simulink model "TestingCleanPPWithStopACC_Brake"  (R2023a)
settings: Solver=FixedStepAuto  StartTime=0.0  StopTime=inf  FixedStep=0.01  RelTol=1e-3
undefined symbols (not defined in the file): accsubsystem_1_data, x, y, z
libraries: mpcsigdimcheck_private x10, ros2lib x7, robotalgslib x1, mpclib x1, drivingvehiclecontroller x1, slpidlib x1
settings Model: Creator=kartosis  LastModifiedBy=almudhaf.3
settings OptimizationCC: EnhancedBackFolding=on  PassReuseOutputArgsAs=Individual arguments  ZeroExternalMemoryAtStartup=off  ZeroInternalMemoryAtStartup=off  MaxStackSize=64  OptimizeBlockOrder=speed  DifferentSizesBufferReuse=on  OptimizationCustomize=off  EfficientTunableParamExpr=on
settings DebuggingCC: ParameterTunabilityLossMsg=error
settings HardwareCC: ProdBitPerLong=64  ProdHWDeviceType=Intel->x86-64 (Linux 64)
settings SFSimCC: MATLABDynamicMemAlloc=off
settings RTWCC: Description=Embedded Coder  SystemTargetFile=ert.tlc  HardwareBoard=Robot Operating System 2 (ROS 2)  TLCOptions="-aInlineSetEventsForThisBaseRateFcn=TLC_FALSE -aSuppressMultiTaskScheduler=TLC_FALSE  -aRateBasedStepFcn=0"  TemplateMakefile=ert_default_tmf  Toolchain=Colcon Tools  TargetLang=C++
settings CodeAppCC: ForceParamTrailComments=on  IgnoreCustomStorageClasses=off  OperatorAnnotations=on  SimulinkDataObjDesc=on  SFDataObjDesc=on  InsertBlockDesc=on
settings ERTTargetCC: CodeInterfacePackaging=C++ class  RootIOFormat=Structure reference

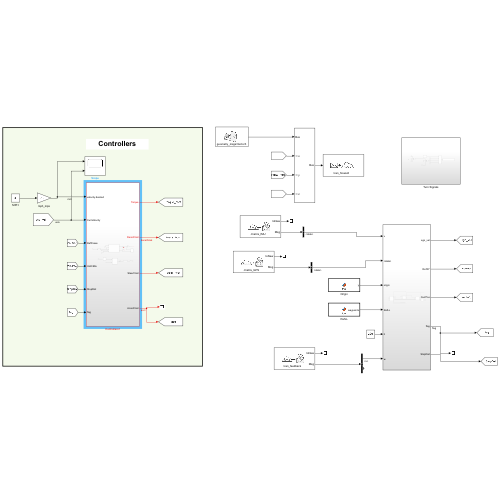
[thumbnail: Simulink's stored preview of the top-level diagram]
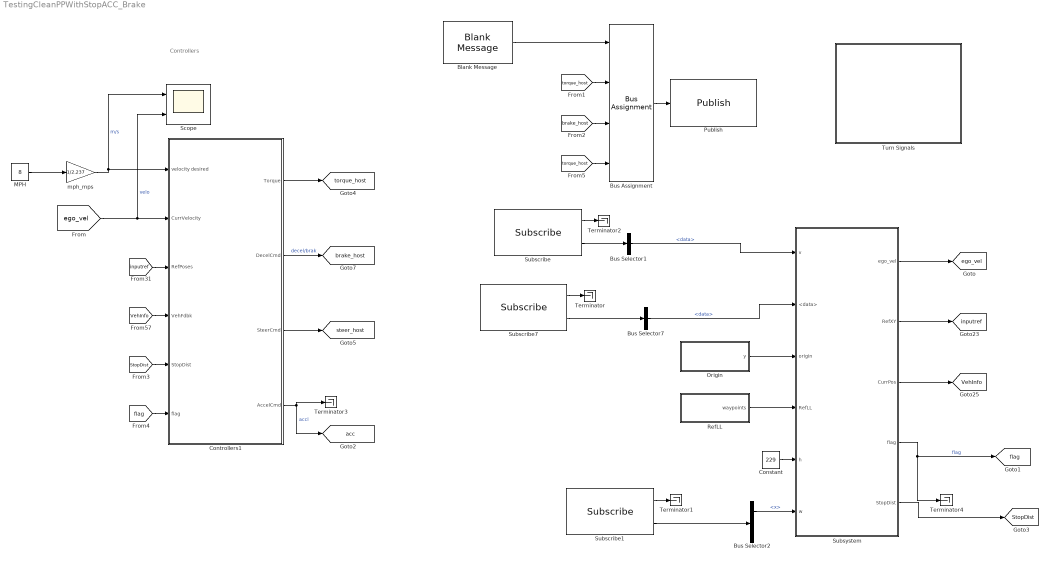
== system TestingCleanPPWithStopACC_Brake ==
  note: Controllers
  Blank Message : ros2lib/Blank Message  messageClass=Message  entityType=geometry_msgs/Vector3  messageType=geometry_msgs/Vector3  SampleTime=0.01
      settings: LibrarySourceBlock=roslib/ROS 2/Blank Message
  Bus Assignment : BusAssignment  AssignedSignals=x,y,z
  Bus Selector1 : BusSelector  OutputSignals=data
  Bus Selector2 : BusSelector  OutputSignals=x,y
  Bus Selector7 : BusSelector  OutputSignals=data
  Constant : Constant  Value=229
  Controllers1 : Subsystem
  MPH : Constant  Value=8
  Origin : MATLAB Function  TreatAsAtomicUnit=on
  Publish : ros2lib/Publish  topicSource=Select from ROS network  topic=/can_forward  messageType=geometry_msgs/Vector3  QOSHistory=Keep last  QOSDepth=1  QOSReliability=Reliable  QOSDurability=Volatile
      settings: LibrarySourceBlock=roslib/ROS 2/Publish
  RefLL : MATLAB Function  TreatAsAtomicUnit=on
  Scope : Scope  NumInputPorts=2
  Subscribe : ros2lib/Subscribe  topicSource=Select from ROS network  topic=/matrix_IMU  messageType=std_msgs/Float64MultiArray  sampleTime=-1  QOSHistory=Keep all  QOSDepth=1  QOSReliability=Reliable  QOSDurability=Volatile
      settings: LibrarySourceBlock=roslib/ROS 2/Subscribe
  Subscribe1 : ros2lib/Subscribe  topicSource=Specify your own  topic=/can_feedback  messageType=geometry_msgs/Vector3  sampleTime=-1  QOSHistory=Keep all  QOSDepth=1  QOSReliability=Reliable  QOSDurability=Volatile
      settings: LibrarySourceBlock=roslib/ROS 2/Subscribe
  Subscribe7 : ros2lib/Subscribe  topicSource=Specify your own  topic=/matrix_GPS  messageType=std_msgs/Float64MultiArray  sampleTime=-1  QOSHistory=Keep all  QOSDepth=1  QOSReliability=Reliable  QOSDurability=Volatile
      settings: LibrarySourceBlock=roslib/ROS 2/Subscribe
  Subsystem : Subsystem
  Terminator{,1..4} (5 alike) : Terminator
  Turn Signals : Subsystem
  mph_mps : Gain  Gain=1/2.237
  tag scope: StopDist=global, VehInfo=global, acc=global, brake_host=global, ego_vel=global, flag=global, inputref=global, steer_host=global, torque_host=global
  wires:
  Blank Message/1 -> Bus Assignment/1
  Bus Assignment/1 -> Publish/1
  Controllers1/1(Torque) -> [torque_host]
  [inputref] -> Controllers1/3(RefPoses)
  [VehInfo] -> Controllers1/4(VehFdbk)
  Controllers1/2(DecelCmd) -> [brake_host]  "decel/brak"
  Controllers1/3(SteerCmd) -> [steer_host]
  Subscribe7/2 -> Bus Selector7/1
  Bus Selector7/1 -> Subsystem/2(<data>)  "<data>"
  Origin/1(y) -> Subsystem/3(origin)
  RefLL/1(waypoints) -> Subsystem/4(RefLL)
  Constant/1 -> Subsystem/5(h)
  Subsystem/1(ego_vel) -> [ego_vel]
  Subsystem/2(RefXY) -> [inputref]
  Bus Selector1/1 -> Subsystem/1(v)  "<data>"
  Subscribe7/1 -> Terminator/1
  Subscribe/2 -> Bus Selector1/1
  Subscribe/1 -> Terminator2/1
  Subsystem/3(CurrPos) -> [VehInfo]
  [ego_vel] -> Controllers1/2(CurrVelocity), Scope/2  "velo"
  mph_mps/1 -> Scope/1, Controllers1/1(velocity desired)  "m/s"
  Subscribe1/1 -> Terminator1/1
  Subscribe1/2 -> Bus Selector2/1
  Bus Selector2/1 -> Subsystem/6(w)  "<x>"
  Controllers1/4(AccelCmd) -> Terminator3/1, [acc]  "accl"
  Subsystem/4(flag) -> Terminator4/1, [flag]  "flag"
  MPH/1 -> mph_mps/1
  [torque_host] -> Bus Assignment/2
  Subsystem/5(StopDist) -> [StopDist]
  [StopDist] -> Controllers1/5(StopDist)
  [flag] -> Controllers1/6(flag)
  [torque_host] -> Bus Assignment/4
  [brake_host] -> Bus Assignment/3

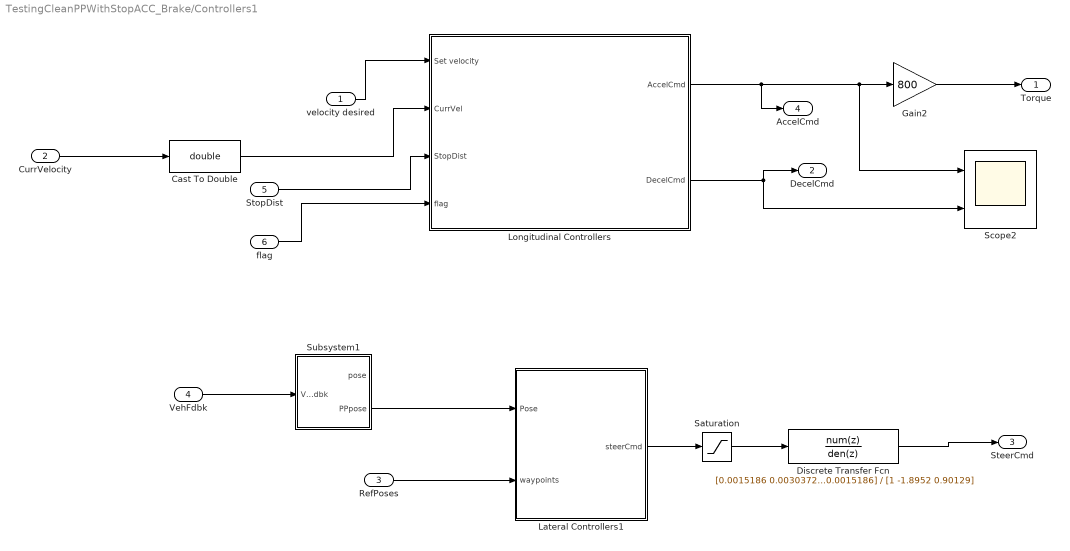
== system TestingCleanPPWithStopACC_Brake/Controllers1 ==
  velocity desired : Inport
  CurrVelocity : Inport  Port=2
  RefPoses : Inport  Port=3
  VehFdbk : Inport  Port=4
  StopDist : Inport  Port=5
  flag : Inport  Port=6
  Cast To Double : DataTypeConversion  OutDataTypeStr=double  SaturateOnIntegerOverflow=off  RndMeth=Floor
  Discrete Transfer Fcn : DiscreteTransferFcn  Numerator=[0.0015186 0.0030372 0.0015186]  Denominator=[1 -1.8952 0.90129]  SampleTime=0.01
  Gain2 : Gain  Gain=800
  Lateral Controllers1 : Subsystem
  Longitudinal Controllers : Subsystem
  Saturation : Saturate  UpperLimit=540  LowerLimit=-540  LinearizeAsGain=off
  Scope2 : Scope  NumInputPorts=2
  Subsystem1 : Subsystem
  Torque : Outport
  DecelCmd : Outport  Port=2
  SteerCmd : Outport  Port=3
  AccelCmd : Outport  Port=4
  wires:
  velocity desired/1 -> Longitudinal Controllers/1(Set velocity)
  Longitudinal Controllers/2(DecelCmd) -> DecelCmd/1, Scope2/2
  Longitudinal Controllers/1(AccelCmd) -> Scope2/1, Gain2/1, AccelCmd/1
  CurrVelocity/1 -> Cast To Double/1
  Subsystem1/2(PPpose) -> Lateral Controllers1/1(Pose)
  VehFdbk/1 -> Subsystem1/1(VehFdbk)
  RefPoses/1 -> Lateral Controllers1/2(waypoints)
  Cast To Double/1 -> Longitudinal Controllers/2(CurrVel)
  Saturation/1 -> Discrete Transfer Fcn/1
  Lateral Controllers1/1(steerCmd) -> Saturation/1
  Discrete Transfer Fcn/1 -> SteerCmd/1
  Gain2/1 -> Torque/1
  StopDist/1 -> Longitudinal Controllers/3(StopDist)
  flag/1 -> Longitudinal Controllers/4(flag)

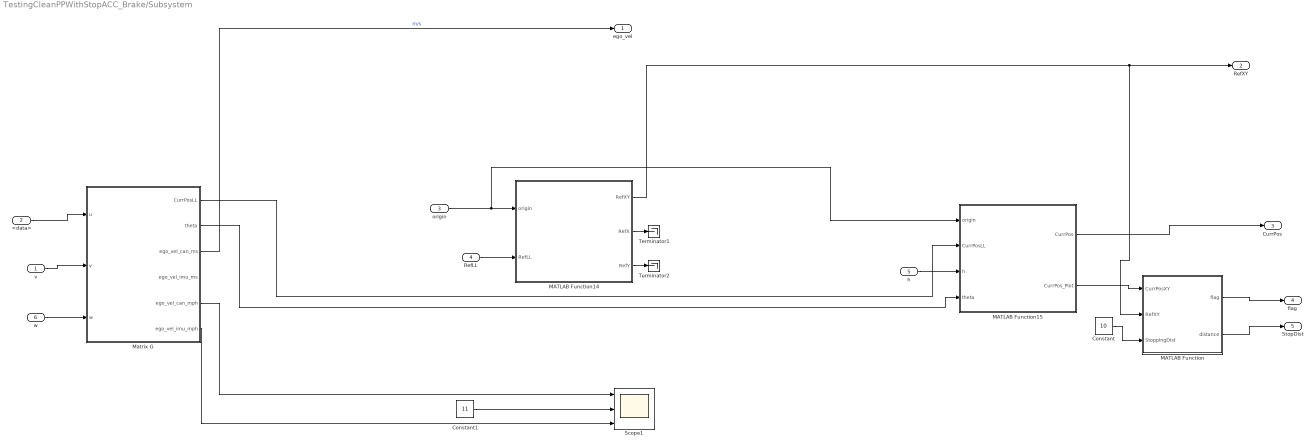
== system TestingCleanPPWithStopACC_Brake/Subsystem ==
  v : Inport
  <data> : Inport  Port=2
  origin : Inport  Port=3
  RefLL : Inport  Port=4
  h : Inport  Port=5
  w : Inport  Port=6
  Constant : Constant  Value=10
  Constant1 : Constant  Value=11
  MATLAB Function : MATLAB Function  TreatAsAtomicUnit=on
  MATLAB Function14 : MATLAB Function  TreatAsAtomicUnit=on
  MATLAB Function15 : MATLAB Function  TreatAsAtomicUnit=on
  Matrix G : MATLAB Function  TreatAsAtomicUnit=on
  Scope1 : Scope  NumInputPorts=3
  Terminator1 : Terminator
  Terminator2 : Terminator
  ego_vel : Outport
  RefXY : Outport  Port=2
  CurrPos : Outport  Port=3
  flag : Outport  Port=4
  StopDist : Outport  Port=5
  wires:
  <data>/1 -> Matrix G/1(u)
  MATLAB Function14/1(RefXY) -> MATLAB Function/2(RefXY), RefXY/1
  MATLAB Function14/3(RefY) -> Terminator2/1
  Matrix G/3(ego_vel_can_ms) -> ego_vel/1  "m/s"
  origin/1 -> MATLAB Function15/1(origin), MATLAB Function14/1(origin)
  Matrix G/2(theta) -> MATLAB Function15/4(theta)
  MATLAB Function15/1(CurrPos) -> CurrPos/1
  RefLL/1 -> MATLAB Function14/2(RefLL)
  h/1 -> MATLAB Function15/3(h)
  Matrix G/1(CurrPosLL) -> MATLAB Function15/2(CurrPosLL)
  MATLAB Function14/2(RefX) -> Terminator1/1
  v/1 -> Matrix G/2(v)
  w/1 -> Matrix G/3(w)
  Constant1/1 -> Scope1/2
  MATLAB Function/1(flag) -> flag/1
  MATLAB Function15/2(CurrPos_Plot) -> MATLAB Function/1(CurrPosXY)
  Matrix G/5(ego_vel_can_mph) -> Scope1/1
  Matrix G/6(ego_vel_imu_mph) -> Scope1/3
  Constant/1 -> MATLAB Function/3(StoppingDist)
  MATLAB Function/2(distance) -> StopDist/1

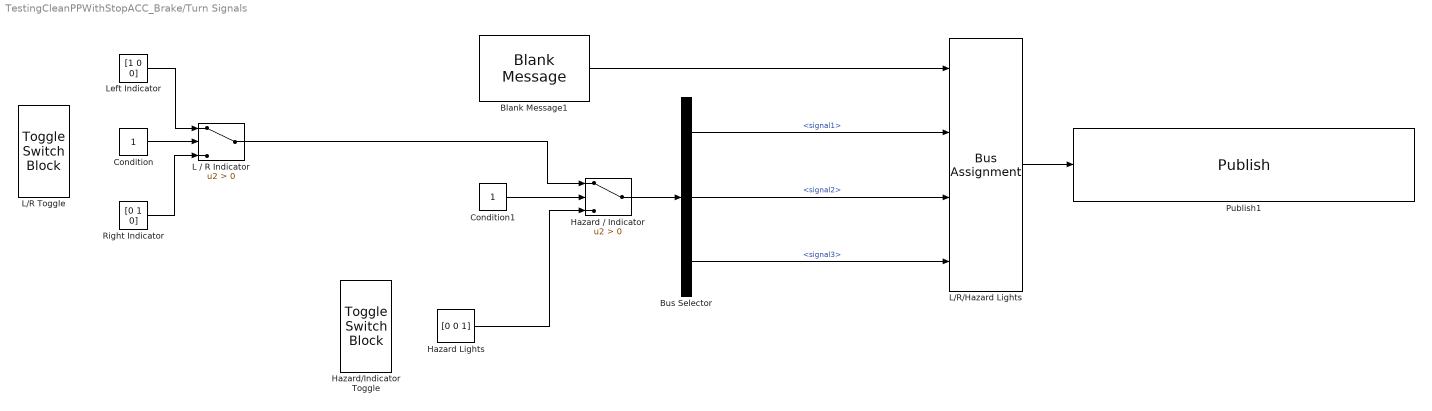
== system TestingCleanPPWithStopACC_Brake/Turn Signals ==
  Blank Message1 : ros2lib/Blank Message  messageClass=Message  entityType=geometry_msgs/Vector3  messageType=geometry_msgs/Vector3  SampleTime=0.01
      settings: LibrarySourceBlock=roslib/ROS 2/Blank Message
  Bus Selector : BusSelector  OutputSignals=signal1,signal2,signal3
  Condition : Constant
  Condition1 : Constant
  Hazard / Indicator : Switch  Criteria=u2 > Threshold  AllowDiffInputSizes=on  SaturateOnIntegerOverflow=off  InputSameDT=off
  Hazard Lights : Constant  Value=[0 0 1]
  Hazard/Indicator Toggle : ToggleSwitchBlock
      settings: Values={{'Off', 'On'}, [0 1]}
  L / R Indicator : Switch  Criteria=u2 > Threshold  SaturateOnIntegerOverflow=off  InputSameDT=off
  L/R Toggle : ToggleSwitchBlock
      settings: Values={{'Off', 'On'}, [0 1]}
  L/R/Hazard Lights : BusAssignment  AssignedSignals=x,y,z
  Left Indicator : Constant  Value=[1 0 0]
  Publish1 : ros2lib/Publish  topicSource=Specify your own  topic=/indicator_lights  messageType=geometry_msgs/Vector3  QOSHistory=Keep last  QOSDepth=1  QOSReliability=Reliable  QOSDurability=Volatile
      settings: LibrarySourceBlock=roslib/ROS 2/Publish
  Right Indicator : Constant  Value=[0 1 0]
  wires:
  Bus Selector/2 -> L/R/Hazard Lights/3  "<signal2>"
  Hazard / Indicator/1 -> Bus Selector/1
  Left Indicator/1 -> L / R Indicator/1
  Bus Selector/3 -> L/R/Hazard Lights/4  "<signal3>"
  Condition/1 -> L / R Indicator/2
  Condition1/1 -> Hazard / Indicator/2
  Right Indicator/1 -> L / R Indicator/3
  L/R/Hazard Lights/1 -> Publish1/1
  Hazard Lights/1 -> Hazard / Indicator/3
  Bus Selector/1 -> L/R/Hazard Lights/2  "<signal1>"
  Blank Message1/1 -> L/R/Hazard Lights/1
  L / R Indicator/1 -> Hazard / Indicator/1

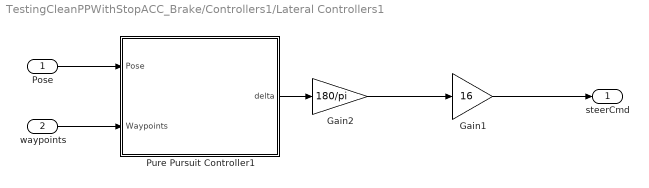
== system TestingCleanPPWithStopACC_Brake/Controllers1/Lateral Controllers1 ==
  Pose : Inport
  waypoints : Inport  Port=2
  Gain1 : Gain  Gain=16
  Gain2 : Gain  Gain=180/pi
  Pure Pursuit Controller1 : Subsystem
  steerCmd : Outport
  wires:
  Pose/1 -> Pure Pursuit Controller1/1(Pose)
  waypoints/1 -> Pure Pursuit Controller1/2(Waypoints)
  Gain2/1 -> Gain1/1
  Gain1/1 -> steerCmd/1
  Pure Pursuit Controller1/1(delta) -> Gain2/1

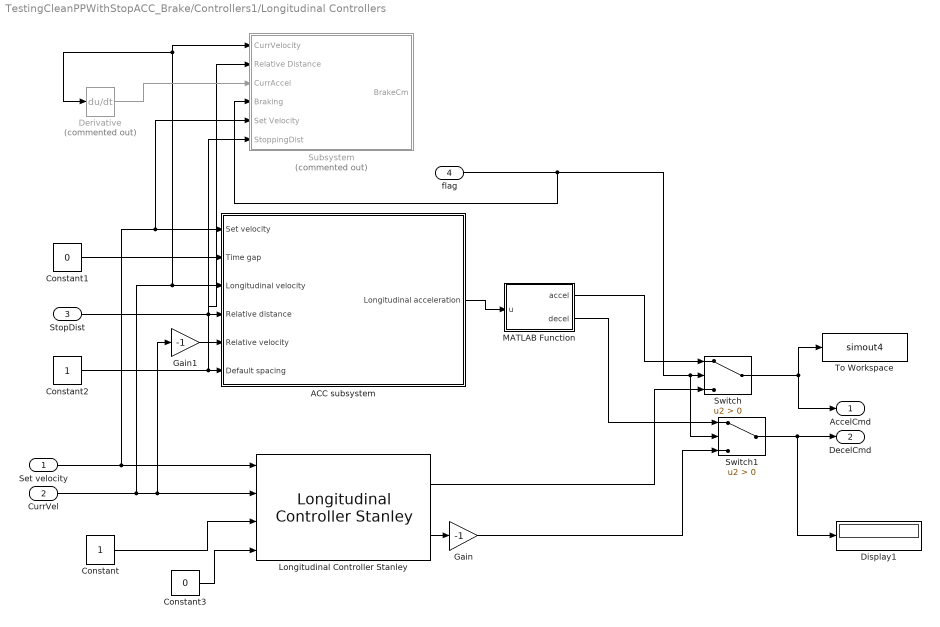
== system TestingCleanPPWithStopACC_Brake/Controllers1/Longitudinal Controllers ==
  Set velocity : Inport
  CurrVel : Inport  Port=2
  StopDist : Inport  Port=3
  flag : Inport  Port=4
  ACC subsystem : Subsystem
      settings: LibrarySourceBlock=mpclib/Automated Driving/Adaptive Cruise Control System
  Constant : Constant
  Constant1 : Constant  Value=0
  Constant2 : Constant
  Constant3 : Constant  Value=0
  Derivative : Derivative  Commented=on
  Display1 : Display
  Gain : Gain  Gain=-1
  Gain1 : Gain  Gain=-1
  Longitudinal Controller Stanley : drivingvehiclecontroller/Longitudinal Controller Stanley  Kp=1.25  Ki=0.12  SampleTime=0.01  MaxAcceleration=2  MaxDeceleration=1.2
  MATLAB Function : MATLAB Function  TreatAsAtomicUnit=on
  Subsystem : Subsystem  Commented=on
  Switch : Switch  Criteria=u2 > Threshold  SaturateOnIntegerOverflow=off  InputSameDT=off
  Switch1 : Switch  Criteria=u2 > Threshold  SaturateOnIntegerOverflow=off  InputSameDT=off
  To Workspace : ToWorkspace  VariableName=simout4  SaveFormat=Timeseries  SampleTime=-1
  AccelCmd : Outport
  DecelCmd : Outport  Port=2
  wires:
  Longitudinal Controller Stanley/2 -> Gain/1
  Set velocity/1 -> Subsystem/5(Set Velocity), ACC subsystem/1(Set velocity), Longitudinal Controller Stanley/1
  Constant3/1 -> Longitudinal Controller Stanley/4
  Constant/1 -> Longitudinal Controller Stanley/3
  CurrVel/1 -> Derivative/1, Subsystem/1(CurrVelocity), ACC subsystem/3(Longitudinal velocity), Gain1/1, Longitudinal Controller Stanley/2
  Constant1/1 -> ACC subsystem/2(Time gap)
  Gain1/1 -> ACC subsystem/5(Relative velocity)
  Constant2/1 -> Subsystem/6(StoppingDist), ACC subsystem/6(Default spacing)
  StopDist/1 -> Subsystem/2(Relative Distance), ACC subsystem/4(Relative distance)
  ACC subsystem/1(Longitudinal acceleration) -> MATLAB Function/1(u)
  flag/1 -> Subsystem/4("Braking "), Switch1/2, Switch/2
  MATLAB Function/1(accel) -> Switch/1
  Longitudinal Controller Stanley/1 -> Switch/3
  Switch/1 -> To Workspace/1, AccelCmd/1
  MATLAB Function/2(decel) -> Switch1/1
  Gain/1 -> Switch1/3
  Switch1/1 -> Display1/1, DecelCmd/1
  Derivative/1 -> Subsystem/3(CurrAccel)

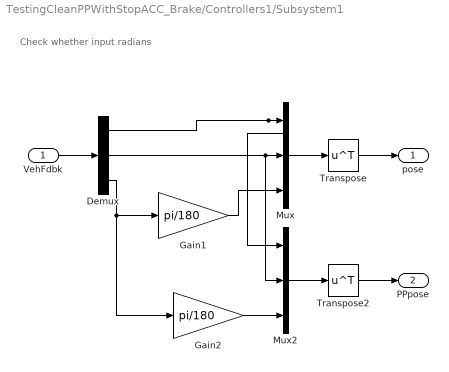
== system TestingCleanPPWithStopACC_Brake/Controllers1/Subsystem1 ==
  note: Check whether input radians
  VehFdbk : Inport
  Demux : Demux  Outputs=3
  Gain1 : Gain  Gain=pi/180
  Gain2 : Gain  Gain=pi/180
  Mux : Mux  Inputs=3
  Mux2 : Mux  Inputs=3
  Transpose : Math  Operator=transpose  SignedPower=on
  Transpose2 : Math  Operator=transpose  SignedPower=on
  pose : Outport
  PPpose : Outport  Port=2
  wires:
  Mux/1 -> Transpose/1
  VehFdbk/1 -> Demux/1
  Gain1/1 -> Mux/3
  Transpose/1 -> pose/1
  Mux2/1 -> Transpose2/1
  Transpose2/1 -> PPpose/1
  Demux/2 -> Mux/2, Mux2/2
  Demux/1 -> Mux2/1, Mux/1
  Demux/3 -> Gain2/1, Gain1/1
  Gain2/1 -> Mux2/3

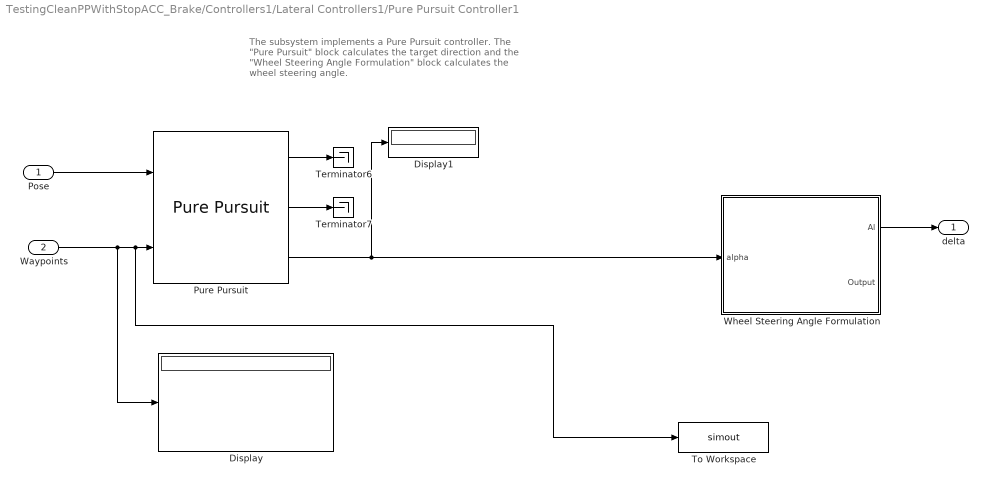
== system TestingCleanPPWithStopACC_Brake/Controllers1/Lateral Controllers1/Pure Pursuit Controller1 ==
  note: The subsystem implements a Pure Pursuit controller. The "Pure Pursuit" block calculates the target direction and the "Wheel Steering Angle Formulation" block calculates the wheel steering angle.
  Pose : Inport
  Waypoints : Inport  Port=2
  Display : Display
  Display1 : Display
  Pure Pursuit : robotalgslib/Pure Pursuit  DesiredLinearVelocity=5  MaxAngularVelocity=1.0  LookaheadDistance=4  TargetDirPort=on  SimulateUsing=Code generation
  Terminator6 : Terminator
  Terminator7 : Terminator
  To Workspace : ToWorkspace  VariableName=simout  SaveFormat=Timeseries  SampleTime=-1
  Wheel Steering Angle Formulation : Subsystem  mask{L=2.865, ld=4}
      mask prompts: L "Bicycle length"; ld "Lookahead distance"
      mask TypeOptions L: Bicycle length/Value
      mask TypeOptions ld: Lookahead distance/Value
      mask Display:
      | image("GeometryMask.png")
      | port_label('input', 1, 'alpha')
      | port_label('output', 1, 'delta')
  delta : Outport
  wires:
  Waypoints/1 -> To Workspace/1, Pure Pursuit/2, Display/1
  Wheel Steering Angle Formulation/1(Al) -> delta/1
  Pure Pursuit/3 -> Wheel Steering Angle Formulation/1(alpha), Display1/1
  Pure Pursuit/2 -> Terminator7/1
  Pose/1 -> Pure Pursuit/1
  Pure Pursuit/1 -> Terminator6/1

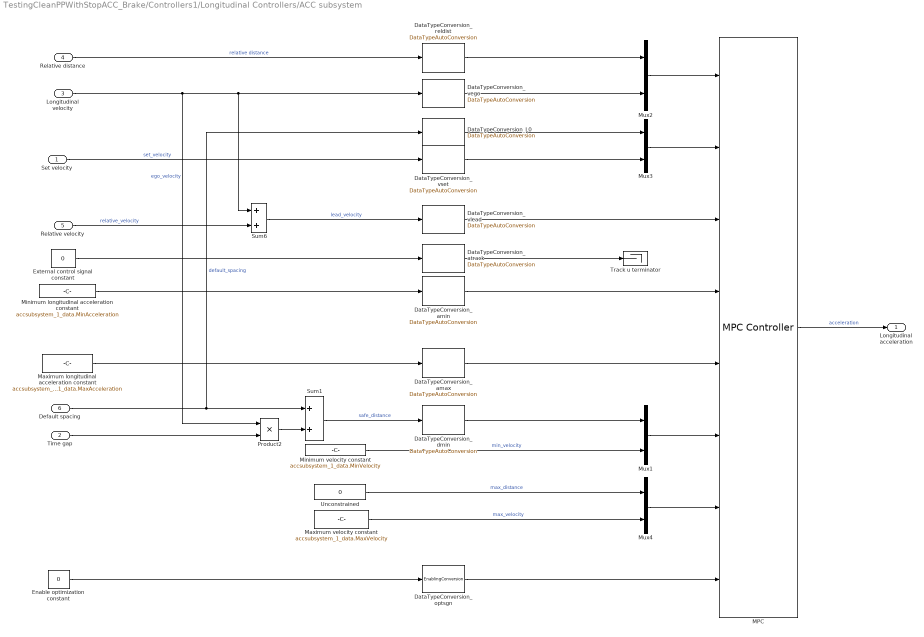
== system TestingCleanPPWithStopACC_Brake/Controllers1/Longitudinal Controllers/ACC subsystem ==
  Set velocity : Inport
  Time gap : Inport  Port=2
  Longitudinal velocity : Inport  Port=3
  Relative distance : Inport  Port=4
  Relative velocity : Inport  Port=5
  Default spacing : Inport  Port=6
  DataTypeConversion_L0 : mpcsigdimcheck_private/DataTypeAutoConversion  datatypestr=accsubsystem_1_data.DataType
      settings: LibrarySourceBlock=mpclib/Automated Driving/Adaptive Cruise Control System/DataTypeConversion_L0
  DataTypeConversion_amax : mpcsigdimcheck_private/DataTypeAutoConversion  datatypestr=accsubsystem_1_data.DataType
      settings: LibrarySourceBlock=mpclib/Automated Driving/Adaptive Cruise Control System/DataTypeConversion_amax
  DataTypeConversion_amin : mpcsigdimcheck_private/DataTypeAutoConversion  datatypestr=accsubsystem_1_data.DataType
      settings: LibrarySourceBlock=mpclib/Automated Driving/Adaptive Cruise Control System/DataTypeConversion_amin
  DataTypeConversion_atrack : mpcsigdimcheck_private/DataTypeAutoConversion  datatypestr=accsubsystem_1_data.DataType
      settings: LibrarySourceBlock=mpclib/Automated Driving/Adaptive Cruise Control System/DataTypeConversion_atrack
  DataTypeConversion_dmin : mpcsigdimcheck_private/DataTypeAutoConversion  datatypestr=accsubsystem_1_data.DataType
      settings: LibrarySourceBlock=mpclib/Automated Driving/Adaptive Cruise Control System/DataTypeConversion_dmin
  DataTypeConversion_optsgn : mpcsigdimcheck_private/EnablingConversion  SystemSampleTime=-1  VariantActivationTime=update diagram  Latency=0  AutoFrameSizeCalculation=off
      settings: LibrarySourceBlock=mpclib/Automated Driving/Adaptive Cruise Control System/DataTypeConversion_optsgn
  DataTypeConversion_reldist : mpcsigdimcheck_private/DataTypeAutoConversion  datatypestr=accsubsystem_1_data.DataType
      settings: LibrarySourceBlock=mpclib/Automated Driving/Adaptive Cruise Control System/DataTypeConversion_reldist
  DataTypeConversion_vego : mpcsigdimcheck_private/DataTypeAutoConversion  datatypestr=accsubsystem_1_data.DataType
      settings: LibrarySourceBlock=mpclib/Automated Driving/Adaptive Cruise Control System/DataTypeConversion_vego
  DataTypeConversion_vlead : mpcsigdimcheck_private/DataTypeAutoConversion  datatypestr=accsubsystem_1_data.DataType
      settings: LibrarySourceBlock=mpclib/Automated Driving/Adaptive Cruise Control System/DataTypeConversion_vlead
  DataTypeConversion_vset : mpcsigdimcheck_private/DataTypeAutoConversion  datatypestr=accsubsystem_1_data.DataType
      settings: LibrarySourceBlock=mpclib/Automated Driving/Adaptive Cruise Control System/DataTypeConversion_vset
  Enable optimization constant : Constant  Value=0  OutDataTypeStr=accsubsystem_1_data.DataType
  External control signal constant : Constant  Value=0  OutDataTypeStr=accsubsystem_1_data.DataType
  MPC : mpclib/MPC Controller  SCDEnableBlockLinearizationSpecification=on  mpcobj=accsubsystem_1_data.Controller  is_multiple=0  enable_value=0  return_u0=off  updateMPCinCallerWorkspace=off  md_inport=on  mv_inport=off  uref_inport=off  return_cost=off  return_mvseq=off  return_qpstatus=off  return_xseq=off  return_state=off  return_ovseq=off  state_inport=off  umin_inport=on  umax_inport=on  ymin_inport=on  ymax_inport=on  cc_inport=off  ywt_inport=off  uwt_inport=off  duwt_inport=off  rhoeps_inport=off  pm_inport=off  MaximumP=10  HorizonChoice=FixedHorizon  n_ts=1  n_p=10  n_mv=1  n_md=2  n_ud=0  n_mo=2  n_uo=0  BlockDataType=double  SampleTimeInherited=off  switch_inport=on
      settings: LibrarySourceBlock=mpclib/Automated Driving/Adaptive Cruise Control System/MPC
  Maximum longitudinal acceleration constant : Constant  Value=accsubsystem_1_data.MaxAcceleration  OutDataTypeStr=accsubsystem_1_data.DataType
  Maximum velocity constant : Constant  Value=accsubsystem_1_data.MaxVelocity  OutDataTypeStr=accsubsystem_1_data.DataType
  Minimum longitudinal acceleration constant : Constant  Value=accsubsystem_1_data.MinAcceleration  OutDataTypeStr=accsubsystem_1_data.DataType
  Minimum velocity constant : Constant  Value=accsubsystem_1_data.MinVelocity  OutDataTypeStr=accsubsystem_1_data.DataType
  Mux{1..4} (4 alike) : Mux  Inputs=[1 1]
  Product2 : Product
  Sum1 : Sum
  Sum6 : Sum
  Track u terminator : Terminator
  Unconstrained : Constant  Value=0  OutDataTypeStr=accsubsystem_1_data.DataType
  Longitudinal acceleration : Outport  PortDimensions=1  VectorParamsAs1DForOutWhenUnconnected=off
  wires:
  DataTypeConversion_atrack/1 -> Track u terminator/1
  External control signal constant/1 -> DataTypeConversion_atrack/1
  DataTypeConversion_optsgn/1 -> MPC/8
  Enable optimization constant/1 -> DataTypeConversion_optsgn/1
  Unconstrained/1 -> Mux4/1  "max_distance"
  Maximum velocity constant/1 -> Mux4/2  "max_velocity"
  Mux4/1 -> MPC/7
  Maximum longitudinal acceleration constant/1 -> DataTypeConversion_amax/1
  Minimum longitudinal acceleration constant/1 -> DataTypeConversion_amin/1
  Set velocity/1 -> DataTypeConversion_vset/1  "set_velocity"
  Time gap/1 -> Product2/2
  DataTypeConversion_vego/1 -> Mux2/2
  DataTypeConversion_reldist/1 -> Mux2/1
  DataTypeConversion_vset/1 -> Mux3/2
  DataTypeConversion_L0/1 -> Mux3/1
  DataTypeConversion_vlead/1 -> MPC/3
  DataTypeConversion_dmin/1 -> Mux1/1
  DataTypeConversion_amin/1 -> MPC/4
  DataTypeConversion_amax/1 -> MPC/5
  Mux1/1 -> MPC/6
  Sum1/1 -> DataTypeConversion_dmin/1  "safe_distance"
  Minimum velocity constant/1 -> Mux1/2  "min_velocity"
  Product2/1 -> Sum1/2
  MPC/1 -> Longitudinal acceleration/1  "acceleration"
  Relative velocity/1 -> Sum6/2  "relative_velocity"
  Relative distance/1 -> DataTypeConversion_reldist/1  "relative distance"
  Longitudinal velocity/1 -> Sum6/1, DataTypeConversion_vego/1, Product2/1  "ego_velocity"
  Mux3/1 -> MPC/2
  Mux2/1 -> MPC/1
  Default spacing/1 -> Sum1/1, DataTypeConversion_L0/1  "default_spacing"
  Sum6/1 -> DataTypeConversion_vlead/1  "lead_velocity"

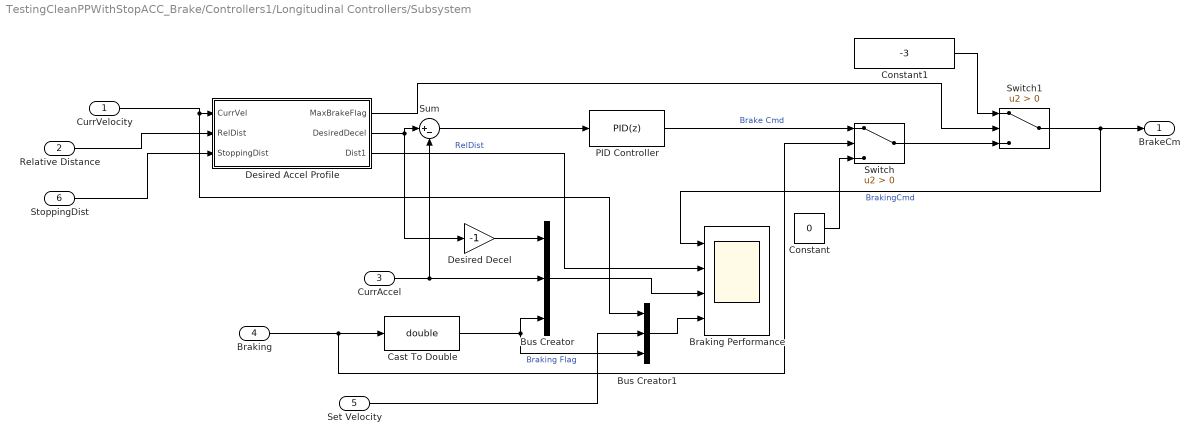
== system TestingCleanPPWithStopACC_Brake/Controllers1/Longitudinal Controllers/Subsystem ==
  CurrVelocity : Inport
  Relative Distance : Inport  Port=2
  CurrAccel : Inport  Port=3
  "Braking " : Inport  Port=4
  Set Velocity : Inport  Port=5
  StoppingDist : Inport  Port=6
  Braking Performance : Scope  NumInputPorts=4
  Bus Creator : BusCreator  Inputs=3
  Bus Creator1 : BusCreator  Inputs=3
  Cast To Double : DataTypeConversion  OutDataTypeStr=double  SaturateOnIntegerOverflow=off  RndMeth=Floor
  Constant : Constant  Value=0
  Constant1 : Constant  Value=-3
  Desired Accel Profile : MATLAB Function  TreatAsAtomicUnit=on
  Desired Decel : Gain  Gain=-1
  PID Controller : slpidlib/PID Controller  Controller=PID  Form=Parallel  TimeDomain=Discrete-time  UseExternalTs=off  SampleTime=0.01  IntegratorMethod=Forward Euler  FilterMethod=Forward Euler  ControllerParametersSource=internal  P=0.05*20  I=0.01*10  UseKiTs=off  D=0  N=100  UseFilter=on  TunerSelectOption=Transfer Function Based (PID Tuner App)  InitialConditionSource=internal  InitialConditionForIntegrator=0  InitialConditionForFilter=0  DifferentiatorICPrevScaledInput=0  ExternalReset=none  TrackingMode=off  Kt=1  LimitOutput=on  SatLimitsSource=internal  UpperSaturationLimit=3  LowerSaturationLimit=-3  LinearizeAsGain=on  AntiWindupMode=none  Kb=1  LimitIntegrator=off  UpperIntegratorSaturationLimit=inf  LowerIntegratorSaturationLimit=-inf  POutMin=[]  POutMax=[]  IOutMin=[]  IOutMax=[]  DOutMin=[]  DOutMax=[]  NOutMin=[]  NOutMax=[]  SumOutMin=[]  SumOutMax=[]  SaturationOutMin=[]  SaturationOutMax=[]  PParamMin=[]  PParamMax=[]  IParamMin=[]  IParamMax=[]  DParamMin=[]  DParamMax=[]  NParamMin=[]  NParamMax=[]  KbParamMin=[]  KbParamMax=[]  KtParamMin=[]  KtParamMax=[]  KbOutMin=[]  KbOutMax=[]  KtOutMin=[]  KtOutMax=[]  IntegratorOutMin=[]  IntegratorOutMax=[]  FilterOutMin=[]  FilterOutMax=[]  SumI1OutMin=[]  SumI1OutMax=[]  SumI2OutMin=[]  SumI2OutMax=[]  SumI3OutMin=[]  SumI3OutMax=[]  SumI4OutMin=[]  SumI4OutMax=[]  SumDOutMin=[]  SumDOutMax=[]  DifferentiatorOutMin=[]  DifferentiatorOutMax=[]  FilterDiffOutCoefMin=[]  FilterDiffOutCoefMax=[]  ReciprocalOutMin=[]  ReciprocalOutMax=[]  SumDenOutMin=[]  SumDenOutMax=[]  SumNumOutMin=[]  SumNumOutMax=[]  DivideOutMin=[]  DivideOutMax=[]  UdiffTsProdOutMin=[]  UdiffTsProdOutMax=[]  NTsProdOutMin=[]  NTsProdOutMax=[]  UintegralTsProdOutMin=[]  UintegralTsProdOutMax=[]  UngainTsProdOutMin=[]  UngainTsProdOutMax=[]  ClampingZeroOutDataTypeStr=Inherit: Inherit via back propagation  ClampingZeroOutMin=[]  ClampingZeroOutMax=[]  FilterDenConstantOutDataTypeStr=Inherit: Inherit via back propagation  FilterDenConstantOutMin=[]  FilterDenConstantOutMax=[]  PCopyOutDataTypeStr=Inherit: Inherit via back propagation  PCopyOutMin=[]  PCopyOutMax=[]  NCopyOutDataTypeStr=Inherit: Inherit via back propagation  NCopyOutMin=[]  NCopyOutMax=[]  IntegratorContinuousStateAttributes=''  IntegratorStateMustResolveToSignalObject=off  IntegratorRTWStateStorageClass=Auto  FilterContinuousStateAttributes=''  FilterStateMustResolveToSignalObject=off  FilterRTWStateStorageClass=Auto  ParallelPVariant=InternalParameters  IdealPVariant=Disabled  IVariant=InternalParameters  DVariant=InternalParameters  IntegratorVariant=Discrete  SatVariant=Enabled  AWVariant=Passthrough  PCopyVariant=Disabled  TRVariant=Disabled  FdbkBlocksVariant=Forward  IdealPFdbkVariant=Disabled  SatFdbkVariant=Disabled  DerivativeFilterVariant=ForwardEulerFilter  NVariant=InternalParameters  NCopyVariant=Disabled  FilterICVariant=InternalICsFilter  IntegratorICVariant=InternalICs  ExternalResetVariant=Disabled  TRSumVariant=Passthrough  SumFdbkVariant=Disabled  SumVariant=Sum_PID  TsampFilterVariant=InternalTs  TsampNgainVariant=Passthrough  TsampIntegralVariant=Disabled_SignalSpec  ExternalSaturationOutDataTypeStr=Inherit: Same as second input
  Sum : Sum  Inputs=|+-
  Switch : Switch  Criteria=u2 > Threshold  SaturateOnIntegerOverflow=off  InputSameDT=off
  Switch1 : Switch  Criteria=u2 > Threshold  SaturateOnIntegerOverflow=off  InputSameDT=off
  BrakeCm : Outport
  wires:
  Relative Distance/1 -> Desired Accel Profile/2(RelDist)
  CurrVelocity/1 -> Bus Creator1/1, Desired Accel Profile/1(CurrVel)
  Sum/1 -> PID Controller/1
  Desired Accel Profile/2(DesiredDecel) -> Sum/1, Desired Decel/1
  "Braking "/1 -> Cast To Double/1, Switch/2
  PID Controller/1 -> Switch/1  "Brake Cmd"
  CurrAccel/1 -> Bus Creator/2, Sum/2
  Desired Decel/1 -> Bus Creator/1
  Constant/1 -> Switch/3
  Switch1/1 -> BrakeCm/1, Braking Performance/1  "BrakingCmd"
  Bus Creator/1 -> Braking Performance/3
  Cast To Double/1 -> Bus Creator1/3, Bus Creator/3  "Braking Flag"
  Desired Accel Profile/3(Dist1) -> Braking Performance/2  "RelDist"
  Switch/1 -> Switch1/3
  Constant1/1 -> Switch1/1
  Desired Accel Profile/1(MaxBrakeFlag) -> Switch1/2
  Bus Creator1/1 -> Braking Performance/4
  Set Velocity/1 -> Bus Creator1/2
  StoppingDist/1 -> Desired Accel Profile/3(StoppingDist)

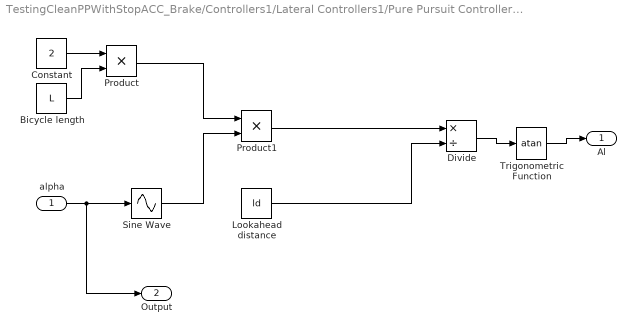
== system TestingCleanPPWithStopACC_Brake/Controllers1/Lateral Controllers1/Pure Pursuit Controller1/Wheel Steering Angle Formulation ==
  alpha : Inport
  Bicycle length : Constant  Value=L
  Constant : Constant  Value=2
  Divide : Product  Inputs=*/
  Lookahead distance : Constant  Value=ld
  Product : Product
  Product1 : Product
  Sine Wave : Sin  TimeSource=Use external signal  SampleTime=0
  Trigonometric Function : Trigonometry  Operator=atan
  Al : Outport
  Output : Outport  Port=2
  wires:
  Sine Wave/1 -> Product1/2
  Bicycle length/1 -> Product/2
  Constant/1 -> Product/1
  Product1/1 -> Divide/1
  Product/1 -> Product1/1
  Divide/1 -> Trigonometric Function/1
  Trigonometric Function/1 -> Al/1
  alpha/1 -> Output/1, Sine Wave/1
  Lookahead distance/1 -> Divide/2

== matlab function TestingCleanPPWithStopACC_Brake/RefLL ==
  data: waypoints output
function waypoints = fcn()


waypoints = [39.99806227837	-83.03238507155	229
39.99806225176	-83.03238507514	229
39.9980622151	-83.03238507952	229
39.99806216774	-83.03238508483	229
39.99806210916	-83.0323850914	229
39.9980620386	-83.03238509932	229
39.99806195496	-83.03238510834	229
39.99806185794	-83.03238511771	229
39.99806174741	-83.03238512699	229
39.99806162342	-83.03238513722	229
39.99806148606	-83.03238514889	229
39.9980613351	-83.03238516134	229
39.99806117106	-83.03238517433	229
39.99806099373	-83.03238518809	229
39.99806080287	-83.03238520311	229
39.99806059877	-83.03238521974	229
39.9980603816	-83.03238523758	229
39.99806015088	-83.03238525624	229
39.99805990597	-83.03238527514	229
39.99805964671	-83.03238529435	229
39.99805937279	-83.03238531348	229
39.99805908445	-83.03238533236	229
39.99805878124	-83.03238535135	229
39.99805846301	-83.0323853721	229
39.99805813043	-83.03238539447	229
39.99805778345	-83.03238541821	229
39.99805742217	-83.03238544562	229
39.99805704525	-83.03238547719	229
39.99805665066	-83.03238551184	229
39.99805623779	-83.03238554698	229
39.99805580651	-83.03238558132	229
39.99805535566	-83.03238561318	229
39.99805488245	-83.03238564368	229
39.99805438579	-83.0323856757	229
39.99805386398	-83.03238570799	229
39.99805331699	-83.03238573957	229
39.99805274668	-83.03238577085	229
39.99805215422	-83.03238580623	229
39.99805153901	-83.03238584858	229
39.99805090072	-83.03238589397	229
39.99805023847	-83.03238593501	229
39.99804955387	-83.0323859732	229
39.99804884854	-83.03238600929	229
39.99804812134	-83.03238604341	229
39.99804736942	-83.03238607335	229
39.99804659222	-83.03238609894	229
39.99804579135	-83.03238612215	229
39.99804496763	-83.0323861475	229
39.99804412175	-83.03238617519	229
39.99804325484	-83.03238620332	229
39.99804236657	-83.032386228	229
39.99804145321	-83.03238625152	229
39.99804051343	-83.032386277	229
39.99803954941	-83.03238630202	229
39.9980385642	-83.03238632304	229
39.9980375606	-83.03238633651	229
39.99803653652	-83.03238634697	229
39.99803548964	-83.03238635868	229
39.99803442351	-83.03238637053	229
39.9980333402	-83.03238638456	229
39.99803223852	-83.03238640484	229
39.99803111484	-83.03238642781	229
39.99802996541	-83.0323864486	229
39.99802879006	-83.03238647172	229
39.99802759101	-83.03238649686	229
39.99802637196	-83.03238652146	229
39.99802513502	-83.03238654417	229
39.99802387934	-83.03238656564	229
39.99802260234	-83.032386585	229
39.99802130181	-83.03238660287	229
39.99801998372	-83.03238661609	229
39.99801864897	-83.0323866234	229
39.99801729425	-83.03238662973	229
39.99801591803	-83.03238663905	229
39.99801452252	-83.03238665271	229
39.99801311009	-83.03238666735	229
39.99801167682	-83.03238667923	229
39.99801021795	-83.03238668921	229
39.99800873742	-83.03238671672	229
39.99800724147	-83.03238675343	229
39.9980057318	-83.03238678991	229
39.99800420585	-83.03238682836	229
39.99800266269	-83.03238687154	229
39.99800110662	-83.032386922	229
39.99799954247	-83.03238697846	229
39.99799796658	-83.03238703209	229
39.99799637829	-83.03238708819	229
39.99799477883	-83.03238714956	229
39.99799317104	-83.0323872162	229
39.99799155708	-83.03238728636	229
39.99798993813	-83.03238735626	229
39.99798831859	-83.03238743124	229
39.99798670493	-83.03238751066	229
39.99798509358	-83.03238761542	229
39.9979834807	-83.0323877503	229
39.99798186778	-83.03238789974	229
39.99798025748	-83.03238805807	229
39.99797865179	-83.03238822672	229
39.99797704903	-83.03238840551	229
39.99797544282	-83.03238859589	229
39.99797383264	-83.03238880248	229
39.99797222769	-83.03238902288	229
39.99797062788	-83.03238924809	229
39.9979690293	-83.03238948477	229
39.99796743185	-83.03238974006	229
39.99796583588	-83.0323900133	229
39.9979642362	-83.03239029449	229
39.99796263389	-83.03239057328	229
39.99796103244	-83.0323908433	229
39.99795942781	-83.03239109745	229
39.99795781729	-83.03239132289	229
39.99795620105	-83.03239152875	229
39.99795457923	-83.03239173027	229
39.99795295492	-83.03239193247	229
39.99795132891	-83.03239214768	229
39.99794969932	-83.03239238496	229
39.99794806376	-83.03239264698	229
39.99794642222	-83.03239292936	229
39.99794478006	-83.03239322594	229
39.99794313768	-83.03239353257	229
39.9979414933	-83.03239384218	229
39.99793984742	-83.03239414331	229
39.99793819886	-83.03239443095	229
39.99793655178	-83.03239470689	229
39.99793491169	-83.03239496597	229
39.99793327721	-83.03239520892	229
39.99793165059	-83.03239545168	229
39.9979300343	-83.03239571043	229
39.99792842977	-83.0323959992	229
39.99792683979	-83.03239632589	229
39.9979252643	-83.03239668805	229
39.99792370386	-83.03239708278	229
39.99792216401	-83.03239751642	229
39.9979206462	-83.0323979888	229
39.99791914359	-83.03239848642	229
39.99791764595	-83.03239900233	229
39.99791615186	-83.03239953319	229
39.99791466259	-83.03240007282	229
39.99791317524	-83.03240062214	229
39.99791169074	-83.03240118781	229
39.99791021889	-83.0324017789	229
39.99790876832	-83.03240240037	229
39.99790734031	-83.03240305497	229
39.9979059366	-83.03240375108	229
39.99790455697	-83.03240449129	229
39.99790319965	-83.03240526838	229
39.9979018623	-83.03240607819	229
39.99790054388	-83.0324069275	229
39.99789924017	-83.03240780389	229
39.99789795049	-83.0324086981	229
39.99789667841	-83.03240961142	229
39.99789542324	-83.03241054286	229
39.99789418065	-83.03241147988	229
39.99789295424	-83.03241244086	229
39.99789174752	-83.03241344165	229
39.99789056469	-83.03241449101	229
39.99788941669	-83.03241558983	229
39.99788830671	-83.03241672758	229
39.99788723077	-83.03241790049	229
39.99788618145	-83.0324191005	229
39.99788515923	-83.0324203259	229
39.99788416924	-83.03242157149	229
39.99788321561	-83.03242283345	229
39.99788229438	-83.03242411282	229
39.99788140433	-83.03242541542	229
39.99788054065	-83.03242674735	229
39.99787969403	-83.03242809984	229
39.99787885465	-83.03242946278	229
39.99787802132	-83.03243083544	229
39.9978772039	-83.03243222385	229
39.99787641925	-83.03243363939	229
39.99787567528	-83.03243508332	229
39.99787496988	-83.0324365466	229
39.99787429569	-83.03243802253	229
39.99787365269	-83.0324395127	229
39.99787304377	-83.03244102356	229
39.99787246485	-83.03244254724	229
39.99787190846	-83.03244407586	229
39.99787137491	-83.03244561086	229
39.99787086386	-83.03244715503	229
39.99787037513	-83.0324487089	229
39.99786991211	-83.03245027402	229
39.99786948354	-83.03245185647	229
39.99786908916	-83.03245345588	229
39.99786871729	-83.03245506829	229
39.9978683647	-83.03245669359	229
39.99786803715	-83.03245833968	229
39.99786773632	-83.03246000806	229
39.99786745744	-83.03246169633	229
39.99786719281	-83.03246340902	229
39.99786693468	-83.03246514706	229
39.99786667599	-83.03246690344	229
39.99786642418	-83.0324686747	229
39.99786618854	-83.03247046119	229
39.99786597319	-83.03247226404	229
39.99786577648	-83.03247408263	229
39.99786560434	-83.03247591964	229
39.99786546061	-83.032477773	229
39.99786534078	-83.03247964459	229
39.99786523319	-83.03248153436	229
39.99786513581	-83.03248343819	229
39.99786504837	-83.03248535536	229
39.99786496749	-83.03248728907	229
39.99786489365	-83.03248923904	229
39.99786481994	-83.03249120448	229
39.99786474423	-83.03249318412	229
39.99786466911	-83.03249517904	229
39.99786459377	-83.032497197	229
39.99786452542	-83.0324992391	229
39.99786447127	-83.03250130323	229
39.99786442322	-83.03250339124	229
39.99786438645	-83.03250549842	229
39.9978643631	-83.03250762136	229
39.99786434627	-83.03250976231	229
39.99786433688	-83.03251192181	229
39.99786434016	-83.03251409964	229
39.99786434669	-83.03251629877	229
39.99786434583	-83.03251852022	229
39.99786434043	-83.03252076373	229
39.99786433301	-83.03252303071	229
39.99786432779	-83.03252532379	229
39.99786432048	-83.03252763963	229
39.99786431669	-83.03252997945	229
39.997864317	-83.03253234028	229
39.99786432461	-83.0325347215	229
39.99786434027	-83.03253712725	229
39.99786436092	-83.03253955137	229
39.9978643841	-83.03254198813	229
39.99786441753	-83.03254444361	229
39.99786445547	-83.03254692468	229
39.99786448592	-83.03254943286	229
39.99786451891	-83.0325519629	229
39.99786455985	-83.03255451664	229
39.99786460762	-83.03255709063	229
39.99786465578	-83.0325596824	229
39.99786470253	-83.03256229242	229
39.99786474797	-83.03256492016	229
39.997864797	-83.03256756004	229
39.99786485285	-83.03257022124	229
39.99786491758	-83.0325729155	229
39.99786499063	-83.03257563502	229
39.99786506073	-83.03257836953	229
39.99786513394	-83.03258112215	229
39.9978652298	-83.03258389599	229
39.99786534595	-83.0325866869	229
39.99786547643	-83.03258949686	229
39.99786561573	-83.032592323	229
39.99786575889	-83.03259517057	229
39.99786589239	-83.03259804605	229
39.99786601256	-83.03260094921	229
39.99786613481	-83.03260387184	229
39.99786625483	-83.03260680408	229
39.99786635896	-83.03260975523	229
39.99786645982	-83.03261271915	229
39.99786657963	-83.03261569892	229
39.99786672562	-83.03261870432	229
39.99786688394	-83.03262173864	229
39.99786705237	-83.03262480073	229
39.99786722844	-83.0326278868	229
39.99786740788	-83.03263099097	229
39.99786758359	-83.03263411042	229
39.99786774092	-83.03263724999	229
39.99786788269	-83.03264040506	229
39.99786802862	-83.03264358187	229
39.99786817869	-83.03264677913	229
39.99786832599	-83.03264999752	229
39.99786847337	-83.03265323294	229
39.99786861926	-83.03265648672	229
39.99786876618	-83.03265976261	229
39.99786891796	-83.03266304875	229
39.99786907453	-83.03266635107	229
39.99786921381	-83.03266967574	229
39.99786935201	-83.03267301512	229
39.9978694976	-83.0326763637	229
39.99786963936	-83.0326797353	229
39.99786978159	-83.0326831261	229
39.99786992807	-83.03268653581	229
39.99787008286	-83.03268995689	229
39.99787024115	-83.0326933889	229
39.99787040459	-83.03269682899	229
39.99787055911	-83.03270026596	229
39.99787070335	-83.03270370666	229
39.99787083062	-83.03270716806	229
39.99787095456	-83.03271064687	229
39.99787108721	-83.032714143	229
39.99787122055	-83.03271764414	229
39.99787135709	-83.03272115129	229
39.99787150799	-83.03272465537	229
39.99787167344	-83.03272815331	229
39.99787184525	-83.03273164835	229
39.99787201876	-83.03273514223	229
39.99787218578	-83.03273863322	229
39.99787234887	-83.03274212339	229
39.997872507	-83.03274560955	229
39.99787265469	-83.03274909034	229
39.9978727989	-83.03275256377	229
39.99787294196	-83.03275603359	229
39.99787308996	-83.03275949873	229
39.99787325072	-83.03276295828	229
39.99787341699	-83.03276641961	229
39.99787359031	-83.03276988277	229
39.9978737753	-83.03277334356	229
39.99787395547	-83.0327767968	229
39.99787412922	-83.0327802426	229
39.99787430473	-83.032783686	229
39.99787447268	-83.03278712923	229
39.99787463889	-83.03279058106	229
39.99787481081	-83.03279403758	229
39.99787498137	-83.03279749736	229
39.99787513555	-83.03280095616	229
39.99787529897	-83.03280441157	229
39.99787547253	-83.0328078565	229
39.99787564259	-83.03281129366	229
39.99787581239	-83.03281472407	229
39.99787598214	-83.03281815266	229
39.99787615917	-83.03282157991	229
39.99787633443	-83.03282501003	229
39.997876504	-83.03282844137	229
39.99787665183	-83.03283187843	229
39.99787678621	-83.0328353223	229
39.99787690553	-83.03283877621	229
39.99787700362	-83.03284224674	229
39.99787710454	-83.03284570243	229
39.99787722889	-83.03284914005	229
39.99787737277	-83.03285256078	229
39.99787754622	-83.03285593517	229
39.99787775435	-83.03285926456	229
39.99787796498	-83.03286256525	229
39.99787815027	-83.0328658544	229
39.99787829223	-83.03286915045	229
39.99787838531	-83.03287245045	229
39.99787846441	-83.03287576495	229
39.99787855093	-83.03287909401	229
39.99787865153	-83.0328824333	229
39.99787877206	-83.03288578091	229
39.99787892839	-83.03288914376	229
39.99787910768	-83.03289251268	229
39.99787928706	-83.03289586935	229
39.99787945725	-83.03289919619	229
39.99787961115	-83.03290248163	229
39.99787975154	-83.03290573283	229
39.99787988006	-83.03290895257	229
39.99787999759	-83.03291214074	229
39.99788010287	-83.03291530282	229
39.99788020246	-83.03291844707	229
39.99788031008	-83.03292157926	229
39.99788042845	-83.03292469795	229
39.99788055421	-83.0329278056	229
39.99788067857	-83.03293090416	229
39.99788079995	-83.03293399092	229
39.99788091585	-83.03293705914	229
39.99788101887	-83.03294010748	229
39.99788111836	-83.03294314065	229
39.9978812164	-83.03294615374	229
39.99788131507	-83.03294914031	229
39.99788141671	-83.03295209899	229
39.99788152354	-83.03295502836	229
39.99788163122	-83.03295793483	229
39.99788173483	-83.032960824	229
39.99788183171	-83.03296369253	229
39.99788192688	-83.03296654083	229
39.99788202155	-83.03296937561	229
39.99788211019	-83.03297219477	229
39.99788219431	-83.03297499566	229
39.99788226936	-83.03297778492	229
39.99788234711	-83.03298055729	229
39.9978824267	-83.03298330655	229
39.99788251289	-83.03298604418	229
39.99788260383	-83.03298876948	229
39.99788269838	-83.0329914781	229
39.99788279279	-83.03299417311	229
39.99788289181	-83.03299685754	229
39.99788299047	-83.03299953561	229
39.99788309464	-83.03300220289	229
39.99788319067	-83.03300485837	229
39.9978832776	-83.0330075037	229
39.9978833531	-83.03301014009	229
39.99788343172	-83.03301277377	229
39.997883523	-83.03301540313	229
39.99788362637	-83.03301802093	229
39.99788373601	-83.03302063038	229
39.99788385289	-83.03302323263	229
39.99788397684	-83.033025826	229
39.99788410322	-83.03302840555	229
39.99788423324	-83.03303096782	229
39.997884379	-83.03303352123	229
39.99788453937	-83.03303606523	229
39.99788472008	-83.0330385988	229
39.99788491352	-83.03304111978	229
39.99788511572	-83.03304362706	229
39.99788533631	-83.03304612153	229
39.99788556759	-83.03304860474	229
39.99788580208	-83.03305107576	229
39.99788603797	-83.03305353151	229
39.99788629057	-83.03305596926	229
39.99788656356	-83.03305839293	229
39.99788686596	-83.03306080162	229
39.99788720319	-83.03306318873	229
39.99788758425	-83.03306555317	229
39.99788800982	-83.03306789619	229
39.99788846913	-83.0330702156	229
39.99788895975	-83.03307251081	229
39.9978894882	-83.03307477537	229
39.99789004175	-83.03307701193	229
39.99789060759	-83.03307923302	229
39.99789119466	-83.03308143911	229
39.9978917997	-83.03308362536	229
39.99789243819	-83.03308577779	229
39.99789311697	-83.03308788874	229
39.99789383158	-83.03308996098	229
39.99789457783	-83.03309199336	229
39.99789535756	-83.03309398856	229
39.99789617063	-83.03309594832	229
39.9978970196	-83.03309787437	229
39.99789790716	-83.03309976787	229
39.99789882643	-83.03310163111	229
39.99789977376	-83.03310346361	229
39.99790074766	-83.03310526432	229
39.99790175883	-83.03310702871	229
39.9979028024	-83.03310875305	229
39.99790387562	-83.03311043376	229
39.99790498207	-83.03311206504	229
39.99790611695	-83.03311364802	229
39.9979072728	-83.03311519072	229
39.9979084484	-83.03311669781	229
39.99790965004	-83.03311816486	229
39.99791088374	-83.03311958253	229
39.99791216007	-83.0331209383	229
39.99791346646	-83.03312223556	229
39.99791478227	-83.03312348732	229
39.99791611545	-83.03312470168	229
39.99791745116	-83.03312590125	229
39.99791878187	-83.0331270931	229
39.99792011302	-83.03312827139	229
39.99792146624	-83.03312939094	229
39.99792284792	-83.03313043844	229
39.99792425702	-83.03313142056	229
39.99792568904	-83.03313234607	229
39.99792714764	-83.03313320782	229
39.99792862747	-83.03313400374	229
39.99793012073	-83.03313473745	229
39.99793162302	-83.03313540712	229
39.99793312224	-83.03313604962	229
39.99793461765	-83.03313668502	229
39.99793611013	-83.03313731275	229
39.99793761009	-83.03313792638	229
39.99793912891	-83.03313852162	229
39.99794067563	-83.03313907806	229
39.99794224525	-83.03313958283	229
39.99794383514	-83.03314004622	229
39.99794544827	-83.03314047099	229
39.99794707246	-83.03314085094	229
39.99794869321	-83.03314119155	229
39.99795030586	-83.0331415112	229
39.99795191356	-83.03314180174	229
39.99795352515	-83.03314204385	229
39.99795511898	-83.03314228106	229
39.99795669749	-83.03314252003	229
39.99795826182	-83.033142751	229
39.99795981829	-83.03314295867	229
39.9979613758	-83.03314314034	229
39.99796293535	-83.03314327907	229
39.99796448968	-83.03314338648	229
39.99796602727	-83.03314349013	229
39.99796755029	-83.03314356918	229
39.99796905909	-83.03314361556	229
39.99797055151	-83.0331436331	229
39.99797202415	-83.03314364756	229
39.99797347605	-83.03314366565	229
39.99797490889	-83.03314368198	229
39.99797633098	-83.03314369617	229
39.99797774542	-83.03314370501	229
39.99797916297	-83.03314371415	229
39.99798058096	-83.03314372785	229
39.9979819959	-83.03314374817	229
39.99798340386	-83.03314377176	229
39.99798479788	-83.03314378597	229
39.99798616992	-83.03314377511	229
39.99798751466	-83.03314375547	229
39.99798883262	-83.03314376177	229
39.99799012553	-83.03314378954	229
39.99799139171	-83.03314382108	229
39.99799262865	-83.03314385481	229
39.99799383823	-83.033143895	229
39.99799501962	-83.03314393683	229
39.99799617313	-83.03314397614	229
39.99799729941	-83.03314400955	229
39.99799839507	-83.03314403597	229
39.99799945575	-83.03314405617	229
39.99800047752	-83.03314407131	229
39.99800146156	-83.03314408337	229
39.99800240247	-83.03314408821	229
39.99800329694	-83.03314409118	229
39.99800414483	-83.03314409974	229
39.99800494734	-83.03314410921	229
39.99800570452	-83.03314411545	229
39.99800641557	-83.03314412348	229
39.9980070818	-83.03314413749	229
39.99800770564	-83.03314415248	229
39.99800828855	-83.03314416343	229
39.99800882983	-83.03314417035	229
39.99800932807	-83.03314417893	229
39.99800978142	-83.03314419151	229
39.99801018801	-83.0331442104	229
39.99801054765	-83.03314423429	229
39.99801086001	-83.03314426169	229
39.99801112427	-83.03314429153	229
39.99801133939	-83.0331443232	229
39.99801150532	-83.03314435534	229
39.99801162287	-83.03314438663	229
39.99801169404	-83.03314441058	229
39.99801171667	-83.03314442597	229
39.9980116959	-83.03314443909	229
39.99801165091	-83.03314445196	229
39.99801160284	-83.03314446755	229
39.99801155776	-83.03314448591	229
39.99801151995	-83.03314450432	229
];

== matlab function TestingCleanPPWithStopACC_Brake/Origin ==
  data: y output
function y = fcn()

y = [39.99806227837	-83.03238507155	229];

end

== matlab function TestingCleanPPWithStopACC_Brake/Subsystem/MATLAB Function ==
  data: CurrPosXY input; flag output; RefXY input; StoppingDist input; distance output
function [flag, distance] = fcn(CurrPosXY, RefXY, StoppingDist)

    RefXYStop = [RefXY(end,1) RefXY(end,2)];
    
    distance = abs(sqrt((RefXYStop(1) - CurrPosXY(1)).^2 + (RefXYStop(2) - CurrPosXY(2)).^2));
    if distance < StoppingDist
        flag = 1;
    else
        flag = 0;
    end
end

== matlab function TestingCleanPPWithStopACC_Brake/Subsystem/Matrix G ==
  data: u input; CurrPosLL output; theta output; ego_vel_can_ms output; v input; w input; ego_vel_imu_ms output; ego_vel_can_mph output; ego_vel_imu_mph output
function [CurrPosLL, theta, ego_vel_can_ms, ego_vel_imu_ms,ego_vel_can_mph,ego_vel_imu_mph] = fcn(u, v, w)
d = double(u(1:2));
lat = double(d(1));
long = d(2);
CurrPosLL=[lat long];

dstar = double(v(1)); %heading angle wrt north
velo = double(w(1)); %non-driven wheel speed
theta = (dstar(1)); 
ego_vel_can_ms = double(velo(1))*0.27778;  %kmh to m/s
ego_vel_imu_ms = double(v(2));  % m/s
ego_vel_can_mph= ego_vel_can_ms*2.237; %m/s to mph
ego_vel_imu_mph=ego_vel_imu_ms*2.237; %m/s 


end

== matlab function TestingCleanPPWithStopACC_Brake/Subsystem/MATLAB Function14 ==
  data: origin input; RefLL input; RefXY output; RefX output; RefY output
function [RefXY,RefX,RefY]   = XYZenu(origin, RefLL)
%size_points = length(RefLL); %100

%zup = h*ones(size_points, 1); %100x1

%points_new = [RefLL, zup]; 

%latlong_new = points_new; 

%origin_new = latlong_new(1,:)

%origin_new = [origin(1) origin(2) origin(3)]; %1x3

xyz = lla2enu(RefLL, origin,'ellipsoid'); 
RefX = xyz(:,1);
RefY = xyz(:,2);
RefXY = [xyz(:,1) xyz(:,2)];


end

== matlab function TestingCleanPPWithStopACC_Brake/Subsystem/MATLAB Function15 ==
  data: CurrPos output; origin input; CurrPosLL input; h input; theta input; CurrPos_Plot output
function [CurrPos, CurrPos_Plot]  = VehicleCurrent(origin, CurrPosLL, h, theta)
zup = h; 
point_new=[CurrPosLL(1), CurrPosLL(2), zup];

x_enu = lla2enu(point_new, origin, 'ellipsoid');

head = 90 - theta;
if head < -180
   head = head + 360;
elseif abs(head) == 180
   head = abs(head);
end

CurrPos=[x_enu(1) x_enu(2) head];
CurrPos_Plot = [x_enu(1) x_enu(2)];

end

== matlab function TestingCleanPPWithStopACC_Brake/Controllers1/Longitudinal Controllers/MATLAB Function ==
  data: u input; accel output; decel output
function [accel, decel] = fcn(u)
if u > 0
    accel=u; decel=0;
elseif u < 0
    accel=0; decel=u;
else
    accel=0;decel=0;
end

== matlab function TestingCleanPPWithStopACC_Brake/Controllers1/Longitudinal Controllers/Subsystem/Desired Accel Profile ==
  data: MaxBrakeFlag output; CurrVel input; DesiredDecel output; RelDist input; Dist1 output; StoppingDist input
function [MaxBrakeFlag,DesiredDecel,Dist1] = AccelProfile(CurrVel,RelDist,StoppingDist)
% time remaining = (current velocity) / (deceleration).
% desired velocity = (stopping distance - current distance) / time remaining.
Dist1 = RelDist;
Dist = Dist1 - StoppingDist;
if Dist1 <= 2
    MaxBrakeFlag = 1;
    DesiredDecel = 0;
else
    MaxBrakeFlag = 0;
    DesiredDecel = -min((CurrVel^2)/(2*Dist),3);
end
%     Dist = RelDist - (2.6850 + 3);
%     Decel = (CurrVel^2)/(2*Dist);
%     RemainingTime = CurrVel/Decel;
%     DesiredVel = Dist/RemainingTime; % DesiredVel = CurrVel/2
